simulink model "system5"  (R2018b)
settings: Solver=VariableStepAuto  StartTime=0.0  StopTime=20  RelTol=1e-3
libraries: cstblocks x5
settings Model: Creator=Abraham Pérez  LastModifiedBy=Abraham Pérez

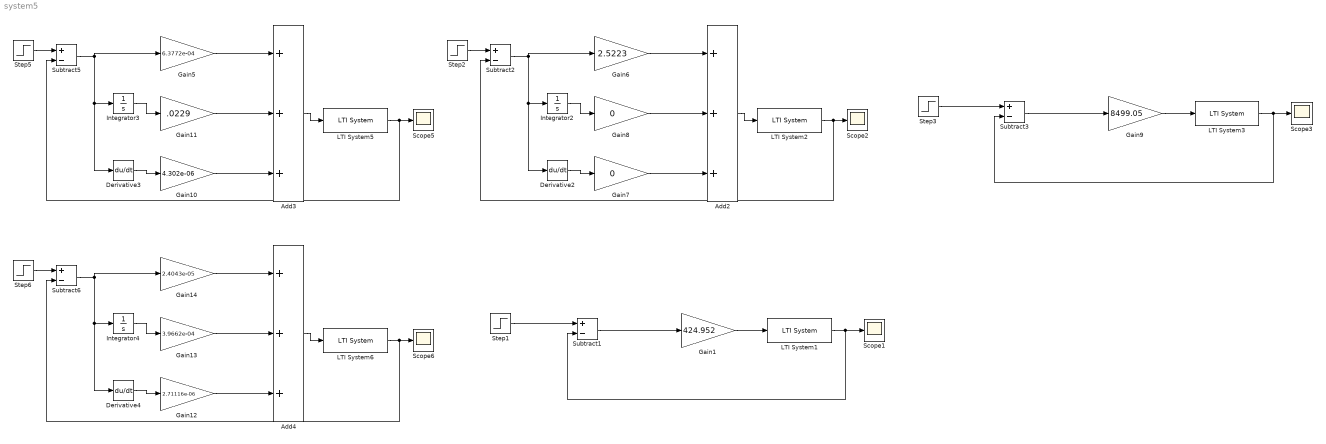
== system system5 ==
  Add2 : Sum  Inputs=+++
  Add3 : Sum  Inputs=+++
  Add4 : Sum  Inputs=+++
  Derivative2 : Derivative
  Derivative3 : Derivative
  Derivative4 : Derivative
  Gain1 : Gain  Gain=424.952
  Gain10 : Gain  Gain=4.302e-06
  Gain11 : Gain  Gain=.0229
  Gain12 : Gain  Gain=2.71116e-06
  Gain13 : Gain  Gain=3.9662e-04
  Gain14 : Gain  Gain=2.4043e-05
  Gain5 : Gain  Gain=6.3772e-04
  Gain6 : Gain  Gain=2.5223
  Gain7 : Gain  Gain=0
  Gain8 : Gain  Gain=0
  Gain9 : Gain  Gain=8499.05
  Integrator2 : Integrator
  Integrator3 : Integrator
  Integrator4 : Integrator
  LTI System1 : cstblocks/LTI System  sys=g5a  IC=[]
  LTI System2 : cstblocks/LTI System  sys=g5b  IC=[]
  LTI System3 : cstblocks/LTI System  sys=g5b  IC=[]
  LTI System5 : cstblocks/LTI System  sys=g5b  IC=[]
  LTI System6 : cstblocks/LTI System  sys=g5a  IC=[]
  Scope{1..3,5..6} (5 alike) : Scope
  Step1 : Step  Time=0  After=10.875  SampleTime=0
  Step2 : Step  Time=0  After=13.775  SampleTime=0
  Step3 : Step  Time=0  After=13.775  SampleTime=0
  Step5 : Step  Time=0  After=13.775  SampleTime=0
  Step6 : Step  Time=0  After=10.875  SampleTime=0
  Subtract{1..3,5..6} (5 alike) : Sum  Inputs=+-
  wires:
  Gain9/1 -> LTI System3/1
  Step3/1 -> Subtract3/1
  LTI System3/1 -> Subtract3/2, Scope3/1
  Gain8/1 -> Add2/2
  Add2/1 -> LTI System2/1
  Integrator2/1 -> Gain8/1
  Gain7/1 -> Add2/3
  Subtract2/1 -> Derivative2/1, Integrator2/1, Gain6/1
  Subtract3/1 -> Gain9/1
  Derivative2/1 -> Gain7/1
  Step2/1 -> Subtract2/1
  LTI System2/1 -> Subtract2/2, Scope2/1
  Gain6/1 -> Add2/1
  Subtract1/1 -> Gain1/1
  LTI System1/1 -> Subtract1/2, Scope1/1
  Step1/1 -> Subtract1/1
  Gain1/1 -> LTI System1/1
  LTI System5/1 -> Subtract5/2, Scope5/1
  Gain5/1 -> Add3/1
  Gain11/1 -> Add3/2
  Derivative3/1 -> Gain10/1
  Integrator3/1 -> Gain11/1
  Step5/1 -> Subtract5/1
  Subtract5/1 -> Derivative3/1, Integrator3/1, Gain5/1
  Gain10/1 -> Add3/3
  Add3/1 -> LTI System5/1
  Add4/1 -> LTI System6/1
  Subtract6/1 -> Derivative4/1, Integrator4/1, Gain14/1
  Step6/1 -> Subtract6/1
  Gain13/1 -> Add4/2
  Gain12/1 -> Add4/3
  Derivative4/1 -> Gain12/1
  Integrator4/1 -> Gain13/1
  Gain14/1 -> Add4/1
  LTI System6/1 -> Subtract6/2, Scope6/1
